simulink model "ES2_1"  (R2022a)
settings: Solver=VariableStepAuto  StartTime=0.0  StopTime=10.0  MaxStep=0.01  RelTol=1e-3
InitFcn:
  | q10=5
  | q20=0
  | q30=0
  | q40=0
  | k1=20;
  | k2=15;
  | m1 =2;
  | m2=1;
  | g=9.8;
  | l=0.5;
settings Model: Creator=Reza  LastModifiedBy=Reza

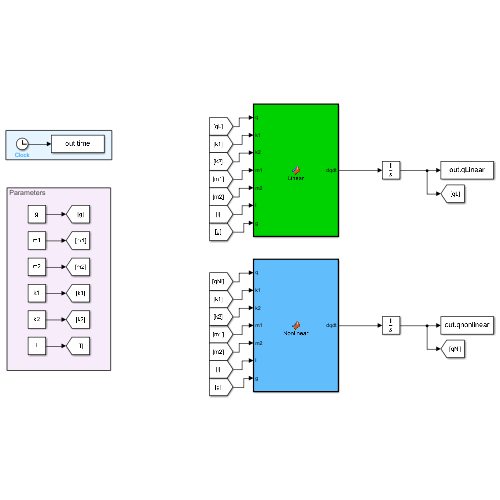
[thumbnail: Simulink's stored preview of the top-level diagram]
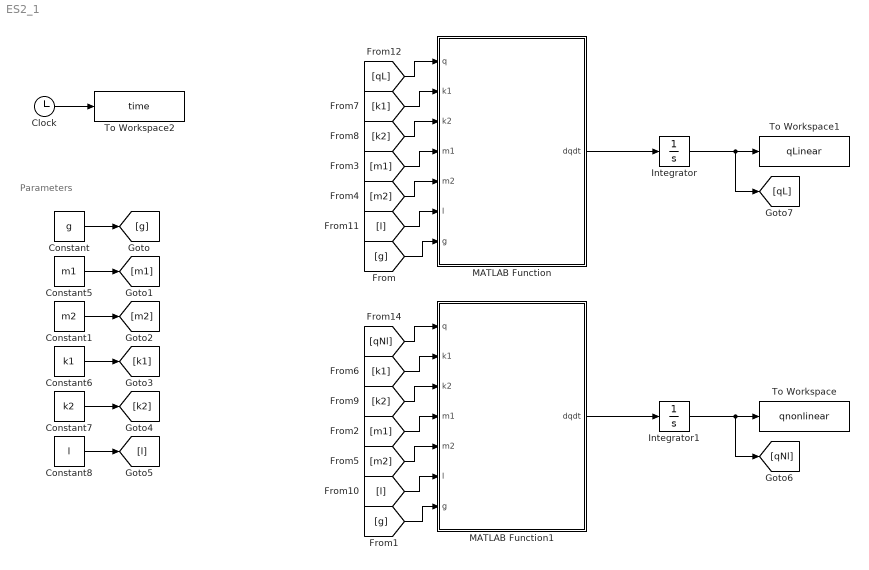
== system ES2_1 ==
  note: Parameters
  Clock : Clock
  Constant : Constant  Value=g
  Constant1 : Constant  Value=m2
  Constant5 : Constant  Value=m1
  Constant6 : Constant  Value=k1
  Constant7 : Constant  Value=k2
  Constant8 : Constant  Value=l
  Integrator : Integrator  InitialCondition=[q10;q20;q30;q40]
  Integrator1 : Integrator  InitialCondition=[q10;q20;q30;q40]
  MATLAB Function : MATLAB Function  TreatAsAtomicUnit=on
  MATLAB Function1 : MATLAB Function  TreatAsAtomicUnit=on
  To Workspace : ToWorkspace  VariableName=qnonlinear  SampleTime=-1
  To Workspace1 : ToWorkspace  VariableName=qLinear  SampleTime=-1
  To Workspace2 : ToWorkspace  VariableName=time  SampleTime=-1
  wires:
  MATLAB Function/1(dqdt) -> Integrator/1
  MATLAB Function1/1(dqdt) -> Integrator1/1
  Constant/1 -> [g]
  [g] -> MATLAB Function/7(g)
  [g] -> MATLAB Function1/7(g)
  Constant5/1 -> [m1]
  [m1] -> MATLAB Function1/4(m1)
  [m1] -> MATLAB Function/4(m1)
  Constant1/1 -> [m2]
  [m2] -> MATLAB Function/5(m2)
  [m2] -> MATLAB Function1/5(m2)
  Constant6/1 -> [k1]
  [k1] -> MATLAB Function1/2(k1)
  [k1] -> MATLAB Function/2(k1)
  Constant7/1 -> [k2]
  [k2] -> MATLAB Function/3(k2)
  [k2] -> MATLAB Function1/3(k2)
  Constant8/1 -> [l]
  [l] -> MATLAB Function1/6(l)
  [l] -> MATLAB Function/6(l)
  Integrator1/1 -> To Workspace/1, [qNl]
  [qNl] -> MATLAB Function1/1(q)
  [qL] -> MATLAB Function/1(q)
  Integrator/1 -> To Workspace1/1, [qL]
  Clock/1 -> To Workspace2/1

== matlab function ES2_1/MATLAB Function1 ==
  data: dqdt output; q input; k1 input; k2 input; m1 input; m2 input; l input; g input
function dqdt = Nonlinear(q,k1,k2,m1,m2,l,g)


dqdt=[q(2);
    -k1*(l*sin(q(1))-l*sin(q(3))*(l*cos(q(1))))/(m1*l^2)-m1*g*l*sin(q(1))/(m1*l^2);
    q(4);
    +k1*(l*sin(q(1))-l*sin(q(3))*(l*cos(q(3))))/(m2*l^2)-k2*(l*sin(q(3)))*(l*cos(q(3)))/(m2*l^2)-m2*g*l*sin(q(3))/(m2*l^2);];
end

== matlab function ES2_1/MATLAB Function ==
  data: dqdt output; q input; k1 input; k2 input; m1 input; m2 input; l input; g input
function dqdt = Linear(q,k1,k2,m1,m2,l,g)


dqdt=[q(2);
    -k1/m1*(q(1)-q(3))-g*q(1)/l;%-k1/m1-g/l*q(1)+k1/m1*q(3);
    q(4);
    k1*(q(1)-q(3))/m2-k2/m2*q(3)-g*q(3)/l;];%k1/m2*q(1)-((k1+k2)/m2+g/l)*q(3)];
end
